simulink model "KF_sim"  (R2016b)
settings: Solver=FixedStepAuto  StartTime=0.0  StopTime=10.0  FixedStep=dt  RelTol=1e-3
values from neighbouring files (symbols this model uses):
  A = [1 dt; 0 1]    [KF_1D.m]    (also in KF_1D_sim.m; KF_3D_if.m = [1]; KF_ex_1.m = [1.9223   -0.9604; KF_free_fall.m = [0 1; 0 0])
  B = [0.5*dt^2 dt]'    [KF_1D.m]    (also in KF_1D_sim.m; KF_3D.m = [1]'; KF_3D_1D.m = [1]'; KF_3D_if.m = [1]')
  C = eye(2)    [KF_1D_sim.m]    (also in KF_ex_1.m = zeros(ObsDim,StateDim); KF_free_fall.m)
  D = [0 0]'    [KF_1D_sim.m]    (also in KF_free_fall.m)
undefined symbols (not defined in the file or in its folder): Discrete, Time
libraries: simulink x1, ctrlSharedLib x1
settings Model: Creator=Daniel  LastModifiedBy=Daniel

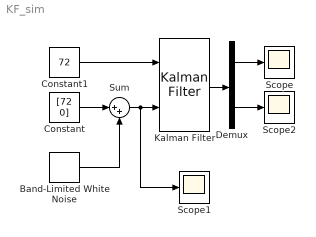
== system KF_sim ==
  Band-Limited White Noise : simulink/Sources/Band-Limited White Noise  Cov=0.001  Ts=0.01  seed=10
  Constant : Constant  Value=[72 0]
  Constant1 : Constant  Value=72
  Demux : Demux  Outputs=2
  Kalman Filter : ctrlSharedLib/Kalman Filter  TimeDomain=Discrete-Time  UseCurrentEstimator=on  ModelSource=Individual A, B, C, D matrices  ModelSourceVariable=ss(0.95,1,1,0,1)  A=A  B=B  C=C  D=D  NumberOfStates=1  NumberOfInputs=1  NumberOfOutputs=1  InitialEstimateSource=Dialog  X0=[80 0]'  P0=10  UseK=off  UseGH=off  NumberOfProcessNoiseInputs=1  G=1  TimeInvariantG=on  H=0  TimeInvariantH=on  Q=0.05  TimeInvariantQ=on  R=1  TimeInvariantR=on  N=0  TimeInvariantN=on  AddInputPort=on  AddEnablePort=off  OutputEstimatedY=off  OutputP=off  Ts=-1
  Scope : Scope
  Scope1 : Scope
  Scope2 : Scope
  Sum : Sum  Inputs=|++
  wires:
  Band-Limited White Noise/1 -> Sum/2
  Constant/1 -> Sum/1
  Sum/1 -> Scope1/1, Kalman Filter/2
  Kalman Filter/1 -> Demux/1
  Constant1/1 -> Kalman Filter/1
  Demux/1 -> Scope/1
  Demux/2 -> Scope2/1
